simulink model "SCHEMA5_SRAX"  (R2023b)
settings: Solver=VariableStepAuto  StartTime=0.0  StopTime=10.0  RelTol=1e-3
values from neighbouring files (symbols this model uses):
  J = (km*ke*Tm)/Ra    (= 0.0225770865363)    [ProiectSACAPCuCalcule.m]
  ke = en/omegaan    (= 0.383940790552)    [ProiectSACAPCuCalcule.m]
  kE = uan/ucn    (= 28.5714285714)    [ProiectSACAPCuCalcule.m]
  kf = (alfa*mn)/omegaan    (= 0.000916591120063)    [ProiectSACAPCuCalcule.m]
  km = mn/ian    (= 0.383940790552)    [ProiectSACAPCuCalcule.m]
  kMI = 3.5/ian    (= 0.7)    [ProiectSACAPCuCalcule.m]
  kMomega = 5/omegaan    (= 0.0238732414638)    [ProiectSACAPCuCalcule.m]
  kr = 1/(2*kPC*Tsuma)    (= 3.51804123711)    [ProiectSACAPCuCalcule.m]
  kxia = 0.008    [ProiectSACAPCuCalcule.m]
  kxw = 0.75    [ProiectSACAPCuCalcule.m]
  ms = mn-mf    (= 1.72773355748)    [ProiectSACAPCuCalcule.m]
  Ra = deltau/ian    (= 3.9175257732)    [ProiectSACAPCuCalcule.m]
  Ta = 0.08    [ProiectSACAPCuCalcule.m]
  Tniu = 0    [ProiectSACAPCuCalcule.m]
  tr = 8.4*Tsuma    (= 0.672)    [ProiectSACAPCuCalcule.m]
  ucn = 3.5    [ProiectSACAPCuCalcule.m]
settings Model: Creator=bartic  LastModifiedBy=bartic

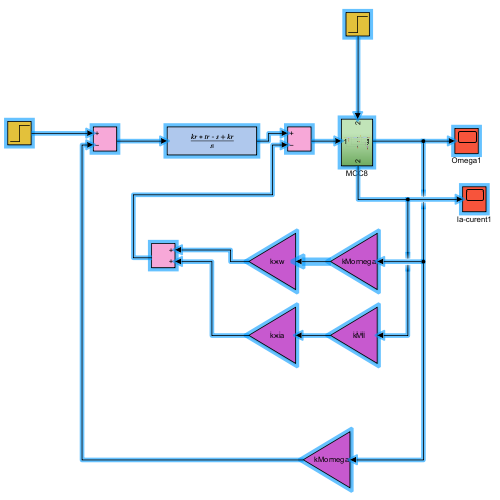
[thumbnail: Simulink's stored preview of the top-level diagram]
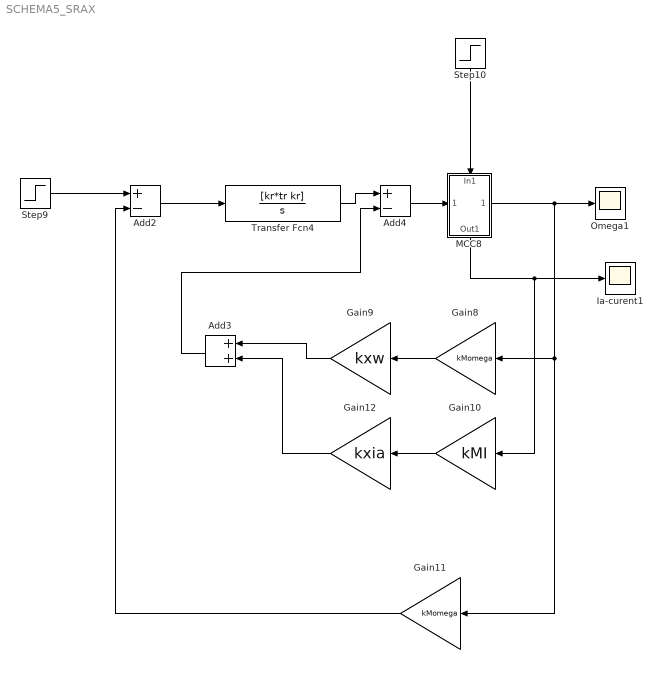
== system SCHEMA5_SRAX ==
  Add2 : Sum  Inputs=+-
  Add3 : Sum
  Add4 : Sum  Inputs=+-
  Gain10 : Gain  Gain=kMI
  Gain11 : Gain  Gain=kMomega
  Gain12 : Gain  Gain=kxia
  Gain8 : Gain  Gain=kMomega
  Gain9 : Gain  Gain=kxw
  Ia-curent1 : Scope
  MCC8 : Subsystem
      settings: PortSchema="{\"entries\":[{\"content\":{\"sides\":[{\"content\":{\"connectorIds\":[\"In1\"]},\"type\":\"ConnectorPlacement.EquallySpacedRectSide\",\"uuid\":\"7f03298a-8e0c-487b-b8a6-e5087a65297a\"},{\"content\":{\"connectorIds\":[\"Out1\"],\"side\":\"RIGHT\"},\"type\":\"ConnectorPlacement.EquallySpacedRectSide\",\"uuid\":\"6b7aaec7-4f5e-4306-aa9a-73fec9d924be\"},{\"content\":{\"connectorIds\":[\"In2\"],\"side\":\"TOP\"},\"type\":\"ConnectorPlacement.EquallySpacedRectSide\",\"uuid\":\"72c2d558-8bfa-4862-bcc5-5bc4cc9947a7\"},{\"content\":{\"connectorIds\":[\"Out2\"],\"side\":\"BOTTOM\"},\"type\":\"ConnectorPlacement.EquallySpacedRectSide\",\"uuid\":\"ddcc37b5-fb8e-4b6e-bf71-41931a3699f4\"}]},\"type\":\"ConnectorPlacement.EquallySpacedConnector\",\"uuid\":\"ed74e97c-0111-4620-8e8b-bcba271a9d3a\"}],\"packageUris\":[\"http://schema.mathworks.com/mf0/Connector/R2020b\"],\"version\":\"1.0\"}"
  Omega1 : Scope
  Step10 : Step  Time=0  After=ms  SampleTime=0
  Step9 : Step  Time=0  After=ucn  SampleTime=0
  Transfer Fcn4 : TransferFcn  Numerator=[kr*tr kr]  Denominator=[1 0]
  wires:
  Add3/1 -> Add4/2
  Gain12/1 -> Add3/2
  Gain9/1 -> Add3/1
  Transfer Fcn4/1 -> Add4/1
  Add4/1 -> MCC8/1(In2)
  Gain11/1 -> Add2/2
  Step9/1 -> Add2/1
  Step10/1 -> MCC8/2(In1)
  Gain10/1 -> Gain12/1
  MCC8/2(Out1) -> Gain10/1, Ia-curent1/1
  Add2/1 -> Transfer Fcn4/1
  MCC8/1(Out2) -> Gain11/1, Gain8/1, Omega1/1
  Gain8/1 -> Gain9/1

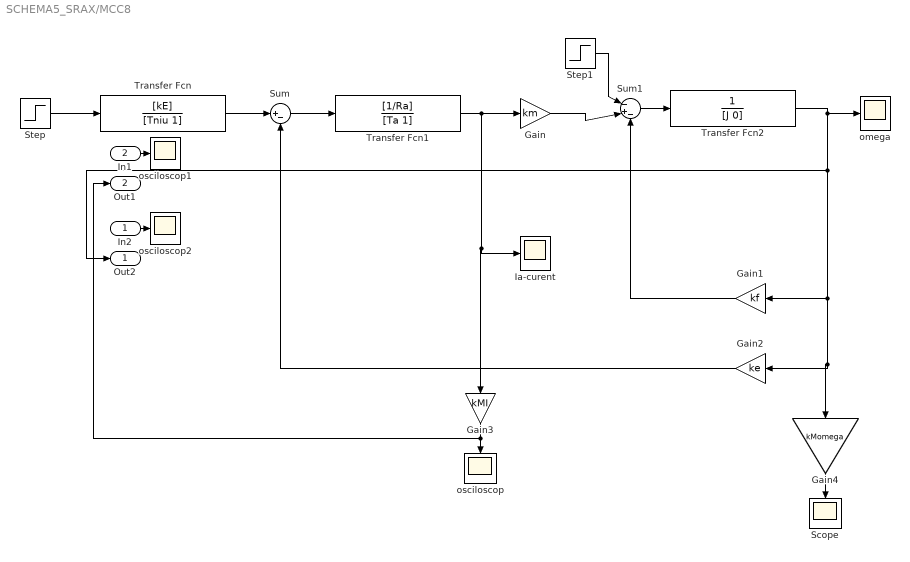
== system SCHEMA5_SRAX/MCC8 ==
  In2 : Inport
  In1 : Inport  Port=2
  Gain : Gain  Gain=km
  Gain1 : Gain  Gain=kf
  Gain2 : Gain  Gain=ke
  Gain3 : Gain  Gain=kMI
  Gain4 : Gain  Gain=kMomega
  Ia-curent : Scope
  Scope : Scope
  Step : Step  Time=0  After=ucn  SampleTime=0
  Step1 : Step  Time=7  After=ms  SampleTime=0
  Sum : Sum  Inputs=|+-
  Sum1 : Sum  Inputs=|-+-
  Transfer Fcn : TransferFcn  Numerator=[kE]  Denominator=[Tniu 1]
  Transfer Fcn1 : TransferFcn  Numerator=[1/Ra]  Denominator=[Ta 1]
  Transfer Fcn2 : TransferFcn  Denominator=[J 0]
  omega : Scope
  osciloscop : Scope
  osciloscop1 : Scope
  osciloscop2 : Scope
  Out2 : Outport
  Out1 : Outport  Port=2
  wires:
  Transfer Fcn2/1 -> Out2/1, Gain4/1, Gain2/1, Gain1/1, omega/1
  Transfer Fcn/1 -> Sum/1
  Sum/1 -> Transfer Fcn1/1
  Transfer Fcn1/1 -> Gain3/1, Ia-curent/1, Gain/1
  Step/1 -> Transfer Fcn/1
  Gain/1 -> Sum1/2
  Step1/1 -> Sum1/1
  Sum1/1 -> Transfer Fcn2/1
  Gain3/1 -> Out1/1, osciloscop/1
  Gain1/1 -> Sum1/3
  Gain4/1 -> Scope/1
  Gain2/1 -> Sum/2
  In1/1 -> osciloscop1/1
  In2/1 -> osciloscop2/1
